simulink model "GTA_PCMFirmware"  (Simulink 7.8)
settings: Solver=FixedStepDiscrete  StartTime=0.0  StopTime=10.0  RelTol=1e-3
PreLoadFcn:
  | try, eval([bdroot '_setup']); catch, eval('model_setup', ''); end
InitFcn:
  | try, eval([bdroot '_setup']); catch, eval('model_setup', ''); end
undefined symbols (not defined in the file): fndFwd, fndNeut, fndRev, FWDlockout, GCM, keySwIgn2, motohawk_build_version, motohawk_trunc_name, motohawk_vardec_path, REVlockout
libraries: MotoHawk_lib x313, simulink x47, GTA_Library x13
(part 4 of 7)

== system GTA_PCMFirmware/Function/1 Inputs and Paramaters/CAN/ Motor Controller/TemperatureWarnFB ==
  note: TempWarnFdbkOK
  In1 : Inport
  Bus Creator : BusCreator
  Bus Selector : BusSelector  OutputSignals=CANTimeout
  Constant : Constant  Value=0  OutDataTypeStr=single
  Constant1 : Constant  Value=0  OutDataTypeStr=single
  Constant2 : Constant  Value=0  OutDataTypeStr=uint16
  Read CAN Message : MotoHawk_lib/CAN Blocks/Read CAN Message  nam='Isolated_CAN'  bus=-2  msg=CANMSG_TempWarnFB  queue=1  slot=''  valid=off  stale=on  labelwires=off
  Relational Operator : RelationalOperator  OutDataTypeStr=boolean
  Signal Specification : SignalSpecification  OutDataTypeStr=single
  Signal Specification1 : SignalSpecification  OutDataTypeStr=single
  Signal Specification2 : SignalSpecification  OutDataTypeStr=uint16
  Subsystem : GTA_Library/Subsystem
  Subsystem1 : GTA_Library/Subsystem
  Subsystem2 : GTA_Library/Subsystem
  motohawk_override_abs : MotoHawk_lib/Calibration & Probing Blocks/motohawk_override_abs  parent_name='WarningFlags'  parent_val=0  show_more=off  name_source=Use Parameter  parent_read_level=1  parent_override_level=1  view_as=Number  enum_struct={'Disabled', 'Enabled'}  use_help_units=off  parent_help=''  parent_units=''  use_min_max=off  parent_min=-inf  parent_max=inf  use_precision=off  parent_precision=''  parent_gain=1  parent_offset=0  parent_exp=1  use_mototune_group=off  parent_group=motohawk_vardec_path(gcb)
  motohawk_override_abs1 : MotoHawk_lib/Calibration & Probing Blocks/motohawk_override_abs  parent_name='MotorTemp'  parent_val=0  show_more=off  name_source=Use Parameter  parent_read_level=1  parent_override_level=1  view_as=Number  enum_struct={'Disabled', 'Enabled'}  use_help_units=off  parent_help=''  parent_units=''  use_min_max=off  parent_min=-inf  parent_max=inf  use_precision=off  parent_precision=''  parent_gain=1  parent_offset=0  parent_exp=1  use_mototune_group=off  parent_group=motohawk_vardec_path(gcb)
  motohawk_override_abs2 : MotoHawk_lib/Calibration & Probing Blocks/motohawk_override_abs  parent_name='HeatSinkTemp'  parent_val=0  show_more=off  name_source=Use Parameter  parent_read_level=1  parent_override_level=1  view_as=Number  enum_struct={'Disabled', 'Enabled'}  use_help_units=off  parent_help=''  parent_units=''  use_min_max=off  parent_min=-inf  parent_max=inf  use_precision=off  parent_precision=''  parent_gain=1  parent_offset=0  parent_exp=1  use_mototune_group=off  parent_group=motohawk_vardec_path(gcb)
  motohawk_probe1 : MotoHawk_lib/Calibration & Probing Blocks/motohawk_probe  nam='WarningFlags'  show_more=off  name_source=Use Parameter  read_level=1  view_as=Number  enum_struct={'Disabled', 'Enabled'}  vector_style=Wide Row  use_help_units=off  help=''  units=''  use_header_enum=off  row_header_enum={}  col_header_enum={}  use_min_max=off  min_val=-inf  max_val=inf  use_precision=off  precision=''  gain=1  offset=0  exp=1  use_mototune_group=off  mototune_group=motohawk_vardec_path(gcb)
  motohawk_probe2 : MotoHawk_lib/Calibration & Probing Blocks/motohawk_probe  nam='MotorTemp'  show_more=off  name_source=Use Parameter  read_level=1  view_as=Number  enum_struct={'Disabled', 'Enabled'}  vector_style=Wide Row  use_help_units=off  help=''  units=''  use_header_enum=off  row_header_enum={}  col_header_enum={}  use_min_max=off  min_val=-inf  max_val=inf  use_precision=off  precision=''  gain=1  offset=0  exp=1  use_mototune_group=off  mototune_group=motohawk_vardec_path(gcb)
  motohawk_probe3 : MotoHawk_lib/Calibration & Probing Blocks/motohawk_probe  nam='HeatSinkTemp'  show_more=off  name_source=Use Parameter  read_level=1  view_as=Number  enum_struct={'Disabled', 'Enabled'}  vector_style=Wide Row  use_help_units=off  help=''  units=''  use_header_enum=off  row_header_enum={}  col_header_enum={}  use_min_max=off  min_val=-inf  max_val=inf  use_precision=off  precision=''  gain=1  offset=0  exp=1  use_mototune_group=off  mototune_group=motohawk_vardec_path(gcb)
  KinTempWarn : Outport
  wires:
  In1/1 -> Bus Selector/1
  Read CAN Message/1 -> Relational Operator/2
  Bus Selector/1 -> Relational Operator/1, Subsystem/1, Subsystem1/1, Subsystem2/1, Subsystem/2, Subsystem1/2, Subsystem2/2  "<CANTimeout>"
  Read CAN Message/2 -> Signal Specification1/1
  Read CAN Message/3 -> Signal Specification/1
  Read CAN Message/4 -> Signal Specification2/1
  Signal Specification2/1 -> Subsystem2/3
  Signal Specification/1 -> Subsystem1/3
  Signal Specification1/1 -> Subsystem/3
  Constant/1 -> Subsystem/4
  Constant2/1 -> Subsystem2/4
  Constant1/1 -> Subsystem1/4
  Subsystem/1 -> motohawk_override_abs2/1, motohawk_probe3/1
  Subsystem1/1 -> motohawk_override_abs1/1, motohawk_probe2/1
  Subsystem2/1 -> motohawk_override_abs/1, motohawk_probe1/1
  motohawk_override_abs/1 -> Bus Creator/4  "WarningFlags"
  Relational Operator/1 -> Bus Creator/1
  motohawk_override_abs2/1 -> Bus Creator/2  "HeatSinkTemp"
  motohawk_override_abs1/1 -> Bus Creator/3  "MotorTemp"
  Bus Creator/1 -> KinTempWarn/1

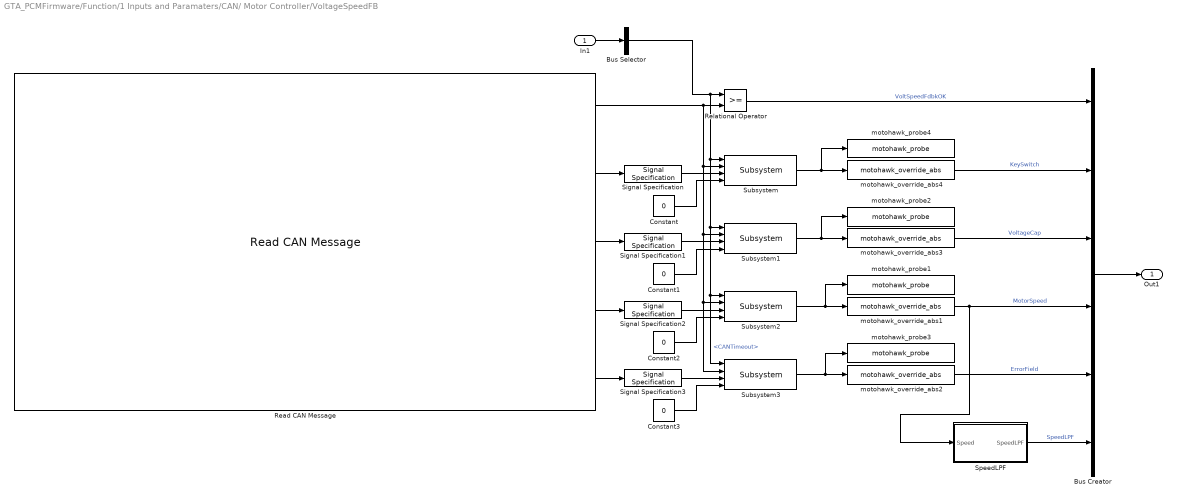
== system GTA_PCMFirmware/Function/1 Inputs and Paramaters/CAN/ Motor Controller/VoltageSpeedFB ==
  In1 : Inport
  Bus Creator : BusCreator  Inputs=6
  Bus Selector : BusSelector  OutputSignals=CANTimeout
  Constant : Constant  Value=0  OutDataTypeStr=single
  Constant1 : Constant  Value=0  OutDataTypeStr=single
  Constant2 : Constant  Value=0  OutDataTypeStr=single
  Constant3 : Constant  Value=0  OutDataTypeStr=uint16
  Read CAN Message : MotoHawk_lib/CAN Blocks/Read CAN Message  nam='Isolated_CAN'  bus=-2  msg=CANMSG_VoltSpeedFB  queue=1  slot=''  valid=off  stale=on  labelwires=off
  Relational Operator : RelationalOperator  OutDataTypeStr=boolean
  Signal Specification : SignalSpecification  OutDataTypeStr=single
  Signal Specification1 : SignalSpecification  OutDataTypeStr=single
  Signal Specification2 : SignalSpecification  OutDataTypeStr=single
  Signal Specification3 : SignalSpecification  OutDataTypeStr=uint16
  SpeedLPF : Subsystem
  Subsystem{,1..3} (4 alike) : GTA_Library/Subsystem
  motohawk_override_abs1 : MotoHawk_lib/Calibration & Probing Blocks/motohawk_override_abs  parent_name='SpeedFiltered'  parent_val=0  show_more=off  name_source=Use Parameter  parent_read_level=1  parent_override_level=1  view_as=Number  enum_struct={'Disabled', 'Enabled'}  use_help_units=off  parent_help=''  parent_units=''  use_min_max=off  parent_min=-inf  parent_max=inf  use_precision=off  parent_precision=''  parent_gain=1  parent_offset=0  parent_exp=1  use_mototune_group=off  parent_group=motohawk_vardec_path(gcb)
  motohawk_override_abs2 : MotoHawk_lib/Calibration & Probing Blocks/motohawk_override_abs  parent_name='ErrorField'  parent_val=0  show_more=off  name_source=Use Parameter  parent_read_level=1  parent_override_level=1  view_as=Number  enum_struct={'Disabled', 'Enabled'}  use_help_units=off  parent_help=''  parent_units=''  use_min_max=off  parent_min=-inf  parent_max=inf  use_precision=off  parent_precision=''  parent_gain=1  parent_offset=0  parent_exp=1  use_mototune_group=off  parent_group=motohawk_vardec_path(gcb)
  motohawk_override_abs3 : MotoHawk_lib/Calibration & Probing Blocks/motohawk_override_abs  parent_name='Voltage_Cap'  parent_val=0  show_more=off  name_source=Use Parameter  parent_read_level=1  parent_override_level=1  view_as=Number  enum_struct={'Disabled', 'Enabled'}  use_help_units=off  parent_help=''  parent_units=''  use_min_max=off  parent_min=-inf  parent_max=inf  use_precision=off  parent_precision=''  parent_gain=1  parent_offset=0  parent_exp=1  use_mototune_group=off  parent_group=motohawk_vardec_path(gcb)
  motohawk_override_abs4 : MotoHawk_lib/Calibration & Probing Blocks/motohawk_override_abs  parent_name='KeySwVoltage'  parent_val=0  show_more=off  name_source=Use Parameter  parent_read_level=1  parent_override_level=1  view_as=Number  enum_struct={'Disabled', 'Enabled'}  use_help_units=off  parent_help=''  parent_units=''  use_min_max=off  parent_min=-inf  parent_max=inf  use_precision=off  parent_precision=''  parent_gain=1  parent_offset=0  parent_exp=1  use_mototune_group=off  parent_group=motohawk_vardec_path(gcb)
  motohawk_probe1 : MotoHawk_lib/Calibration & Probing Blocks/motohawk_probe  nam='SpeedFiltered'  show_more=off  name_source=Use Parameter  read_level=1  view_as=Number  enum_struct={'Disabled', 'Enabled'}  vector_style=Wide Row  use_help_units=off  help=''  units=''  use_header_enum=off  row_header_enum={}  col_header_enum={}  use_min_max=off  min_val=-inf  max_val=inf  use_precision=off  precision=''  gain=1  offset=0  exp=1  use_mototune_group=off  mototune_group=motohawk_vardec_path(gcb)
  motohawk_probe2 : MotoHawk_lib/Calibration & Probing Blocks/motohawk_probe  nam='Voltage_Cap'  show_more=off  name_source=Use Parameter  read_level=1  view_as=Number  enum_struct={'Disabled', 'Enabled'}  vector_style=Wide Row  use_help_units=off  help=''  units=''  use_header_enum=off  row_header_enum={}  col_header_enum={}  use_min_max=off  min_val=-inf  max_val=inf  use_precision=off  precision=''  gain=1  offset=0  exp=1  use_mototune_group=off  mototune_group=motohawk_vardec_path(gcb)
  motohawk_probe3 : MotoHawk_lib/Calibration & Probing Blocks/motohawk_probe  nam='ErrorField'  show_more=off  name_source=Use Parameter  read_level=1  view_as=Number  enum_struct={'Disabled', 'Enabled'}  vector_style=Wide Row  use_help_units=off  help=''  units=''  use_header_enum=off  row_header_enum={}  col_header_enum={}  use_min_max=off  min_val=-inf  max_val=inf  use_precision=off  precision=''  gain=1  offset=0  exp=1  use_mototune_group=off  mototune_group=motohawk_vardec_path(gcb)
  motohawk_probe4 : MotoHawk_lib/Calibration & Probing Blocks/motohawk_probe  nam='KeySwVoltage'  show_more=off  name_source=Use Parameter  read_level=1  view_as=Number  enum_struct={'Disabled', 'Enabled'}  vector_style=Wide Row  use_help_units=off  help=''  units=''  use_header_enum=off  row_header_enum={}  col_header_enum={}  use_min_max=off  min_val=-inf  max_val=inf  use_precision=off  precision=''  gain=1  offset=0  exp=1  use_mototune_group=off  mototune_group=motohawk_vardec_path(gcb)
  Out1 : Outport
  wires:
  In1/1 -> Bus Selector/1
  Read CAN Message/1 -> Relational Operator/2, Subsystem/2, Subsystem1/2, Subsystem2/2, Subsystem3/2
  Bus Selector/1 -> Relational Operator/1, Subsystem/1, Subsystem1/1, Subsystem2/1, Subsystem3/1  "<CANTimeout>"
  Read CAN Message/2 -> Signal Specification/1
  Read CAN Message/5 -> Signal Specification3/1
  Read CAN Message/4 -> Signal Specification2/1
  Read CAN Message/3 -> Signal Specification1/1
  Constant/1 -> Subsystem/4
  Signal Specification/1 -> Subsystem/3
  Signal Specification1/1 -> Subsystem1/3
  Constant1/1 -> Subsystem1/4
  Signal Specification2/1 -> Subsystem2/3
  Constant2/1 -> Subsystem2/4
  Constant3/1 -> Subsystem3/4
  Signal Specification3/1 -> Subsystem3/3
  Subsystem/1 -> motohawk_override_abs4/1, motohawk_probe4/1
  Subsystem1/1 -> motohawk_override_abs3/1, motohawk_probe2/1
  Subsystem2/1 -> motohawk_override_abs1/1, motohawk_probe1/1
  Subsystem3/1 -> motohawk_override_abs2/1, motohawk_probe3/1
  motohawk_override_abs2/1 -> Bus Creator/5  "ErrorField"
  Relational Operator/1 -> Bus Creator/1  "VoltSpeedFdbkOK"
  motohawk_override_abs1/1 -> Bus Creator/4, SpeedLPF/1(Speed)  "MotorSpeed"
  motohawk_override_abs3/1 -> Bus Creator/3  "VoltageCap"
  motohawk_override_abs4/1 -> Bus Creator/2  "KeySwitch"
  SpeedLPF/1(SpeedLPF) -> Bus Creator/6  "SpeedLPF"
  Bus Creator/1 -> Out1/1

== system GTA_PCMFirmware/Function/1 Inputs and Paramaters/CAN/ Motor Controller/Watchdog ==
  In1 : Inport
  Bus Creator : BusCreator  Inputs=2
  Bus Selector : BusSelector  OutputSignals=CANTimeout
  Constant3 : Constant  Value=0  OutDataTypeStr=uint16
  Read CAN Message : MotoHawk_lib/CAN Blocks/Read CAN Message  nam='Isolated_CAN'  bus=-2  msg=CANMSG_Watchdog  queue=1  slot=''  valid=off  stale=on  labelwires=off
  Relational Operator : RelationalOperator  OutDataTypeStr=boolean
  Signal Specification3 : SignalSpecification  OutDataTypeStr=uint16
  Subsystem : GTA_Library/Subsystem
  motohawk_override_abs2 : MotoHawk_lib/Calibration & Probing Blocks/motohawk_override_abs  parent_name='WDcounter'  parent_val=0  show_more=off  name_source=Use Parameter  parent_read_level=1  parent_override_level=1  view_as=Number  enum_struct={'Disabled', 'Enabled'}  use_help_units=off  parent_help=''  parent_units=''  use_min_max=off  parent_min=-inf  parent_max=inf  use_precision=off  parent_precision=''  parent_gain=1  parent_offset=0  parent_exp=1  use_mototune_group=off  parent_group=motohawk_vardec_path(gcb)
  motohawk_probe3 : MotoHawk_lib/Calibration & Probing Blocks/motohawk_probe  nam='WDcounter'  show_more=off  name_source=Use Parameter  read_level=1  view_as=Number  enum_struct={'Disabled', 'Enabled'}  vector_style=Wide Row  use_help_units=off  help=''  units=''  use_header_enum=off  row_header_enum={}  col_header_enum={}  use_min_max=off  min_val=-inf  max_val=inf  use_precision=off  precision=''  gain=1  offset=0  exp=1  use_mototune_group=off  mototune_group=motohawk_vardec_path(gcb)
  KinWatchdog : Outport
  wires:
  In1/1 -> Bus Selector/1
  Constant3/1 -> Subsystem/4
  Signal Specification3/1 -> Subsystem/3
  Read CAN Message/2 -> Signal Specification3/1
  Read CAN Message/1 -> Relational Operator/2, Subsystem/2
  Bus Selector/1 -> Relational Operator/1, Subsystem/1  "<CANTimeout>"
  Relational Operator/1 -> Bus Creator/1  "WatchdogCANok"
  Subsystem/1 -> motohawk_override_abs2/1, motohawk_probe3/1
  motohawk_override_abs2/1 -> Bus Creator/2  "WDcounter"
  Bus Creator/1 -> KinWatchdog/1

== system GTA_PCMFirmware/Function/1 Inputs and Paramaters/CAN/BMS/  Current Sensor ==
  CAN Params : Inport
  Bus Creator : BusCreator  Inputs=6
  Bus Selector : BusSelector  OutputSignals=CANTimeout,MinSOC
  Read CAN Message : MotoHawk_lib/CAN Blocks/Read CAN Message  nam='BMS_CAN'  bus=-2  msg=CANMSG_FluxPowerCurrentSensor  queue=1  slot=''  valid=off  stale=on  labelwires=off
  Relational Operator : RelationalOperator  OutDataTypeStr=boolean
  Signal Specification{,1..3} (4 alike) : SignalSpecification  OutDataTypeStr=single
  UserSOC : Subsystem
  motohawk_override_abs : MotoHawk_lib/Calibration & Probing Blocks/motohawk_override_abs  parent_name='CurrentSensor_Current'  parent_val=0  show_more=off  name_source=Use Parameter  parent_read_level=1  parent_override_level=1  view_as=Number  enum_struct={'Disabled', 'Enabled'}  use_help_units=off  parent_help=''  parent_units=''  use_min_max=off  parent_min=-inf  parent_max=inf  use_precision=off  parent_precision=''  parent_gain=1  parent_offset=0  parent_exp=1  use_mototune_group=off  parent_group=motohawk_vardec_path(gcb)
  motohawk_override_abs1 : MotoHawk_lib/Calibration & Probing Blocks/motohawk_override_abs  parent_name='CurrentSensor_SOC'  parent_val=0  show_more=off  name_source=Use Parameter  parent_read_level=1  parent_override_level=1  view_as=Number  enum_struct={'Disabled', 'Enabled'}  use_help_units=off  parent_help=''  parent_units=''  use_min_max=off  parent_min=-inf  parent_max=inf  use_precision=off  parent_precision=''  parent_gain=1  parent_offset=0  parent_exp=1  use_mototune_group=off  parent_group=motohawk_vardec_path(gcb)
  motohawk_override_abs2 : MotoHawk_lib/Calibration & Probing Blocks/motohawk_override_abs  parent_name='CurrentSensor_Temperature'  parent_val=0  show_more=off  name_source=Use Parameter  parent_read_level=1  parent_override_level=1  view_as=Number  enum_struct={'Disabled', 'Enabled'}  use_help_units=off  parent_help=''  parent_units=''  use_min_max=off  parent_min=-inf  parent_max=inf  use_precision=off  parent_precision=''  parent_gain=1  parent_offset=0  parent_exp=1  use_mototune_group=off  parent_group=motohawk_vardec_path(gcb)
  motohawk_override_abs3 : MotoHawk_lib/Calibration & Probing Blocks/motohawk_override_abs  parent_name='CurrentSensor_AmpHours'  parent_val=0  show_more=off  name_source=Use Parameter  parent_read_level=1  parent_override_level=1  view_as=Number  enum_struct={'Disabled', 'Enabled'}  use_help_units=off  parent_help=''  parent_units=''  use_min_max=off  parent_min=-inf  parent_max=inf  use_precision=off  parent_precision=''  parent_gain=1  parent_offset=0  parent_exp=1  use_mototune_group=off  parent_group=motohawk_vardec_path(gcb)
  motohawk_probe : MotoHawk_lib/Calibration & Probing Blocks/motohawk_probe  nam='CurrentSensor_Current'  show_more=off  name_source=Use Parameter  read_level=1  view_as=Number  enum_struct={'Disabled', 'Enabled'}  vector_style=Wide Row  use_help_units=off  help=''  units=''  use_header_enum=off  row_header_enum={}  col_header_enum={}  use_min_max=off  min_val=-inf  max_val=inf  use_precision=off  precision=''  gain=1  offset=0  exp=1  use_mototune_group=off  mototune_group=motohawk_vardec_path(gcb)
  motohawk_probe1 : MotoHawk_lib/Calibration & Probing Blocks/motohawk_probe  nam='CurrentSensor_SOC'  show_more=off  name_source=Use Parameter  read_level=1  view_as=Number  enum_struct={'Disabled', 'Enabled'}  vector_style=Wide Row  use_help_units=off  help=''  units=''  use_header_enum=off  row_header_enum={}  col_header_enum={}  use_min_max=off  min_val=-inf  max_val=inf  use_precision=off  precision=''  gain=1  offset=0  exp=1  use_mototune_group=off  mototune_group=motohawk_vardec_path(gcb)
  motohawk_probe2 : MotoHawk_lib/Calibration & Probing Blocks/motohawk_probe  nam='CurrentSensor_Temperature'  show_more=off  name_source=Use Parameter  read_level=1  view_as=Number  enum_struct={'Disabled', 'Enabled'}  vector_style=Wide Row  use_help_units=off  help=''  units=''  use_header_enum=off  row_header_enum={}  col_header_enum={}  use_min_max=off  min_val=-inf  max_val=inf  use_precision=off  precision=''  gain=1  offset=0  exp=1  use_mototune_group=off  mototune_group=motohawk_vardec_path(gcb)
  motohawk_probe3 : MotoHawk_lib/Calibration & Probing Blocks/motohawk_probe  nam='CurrentSensor_AmpHours'  show_more=off  name_source=Use Parameter  read_level=1  view_as=Number  enum_struct={'Disabled', 'Enabled'}  vector_style=Wide Row  use_help_units=off  help=''  units=''  use_header_enum=off  row_header_enum={}  col_header_enum={}  use_min_max=off  min_val=-inf  max_val=inf  use_precision=off  precision=''  gain=1  offset=0  exp=1  use_mototune_group=off  mototune_group=motohawk_vardec_path(gcb)
  Current Sensor : Outport
  wires:
  Read CAN Message/1 -> Relational Operator/2
  CAN Params/1 -> Bus Selector/1
  Bus Selector/1 -> Relational Operator/1  "<CANTimeout>"
  Read CAN Message/2 -> Signal Specification/1
  Read CAN Message/3 -> Signal Specification1/1
  Read CAN Message/4 -> Signal Specification2/1
  Read CAN Message/5 -> Signal Specification3/1
  Signal Specification/1 -> motohawk_override_abs/1, motohawk_probe/1
  Signal Specification1/1 -> motohawk_override_abs1/1, motohawk_probe1/1
  Signal Specification2/1 -> motohawk_override_abs2/1, motohawk_probe2/1
  Signal Specification3/1 -> motohawk_override_abs3/1, motohawk_probe3/1
  motohawk_override_abs3/1 -> Bus Creator/5  "csAmpHours"
  motohawk_override_abs2/1 -> Bus Creator/4  "csTemperature"
  motohawk_override_abs1/1 -> Bus Creator/3, UserSOC/1(csSOC)  "csSOC"
  motohawk_override_abs/1 -> Bus Creator/2  "csCurrent"
  Relational Operator/1 -> Bus Creator/1  "csCANok"
  Bus Creator/1 -> Current Sensor/1
  Bus Selector/2 -> UserSOC/2(MinSOC)  "<MinSOC>"
  UserSOC/1(UserSOC) -> Bus Creator/6  "UserSOC"

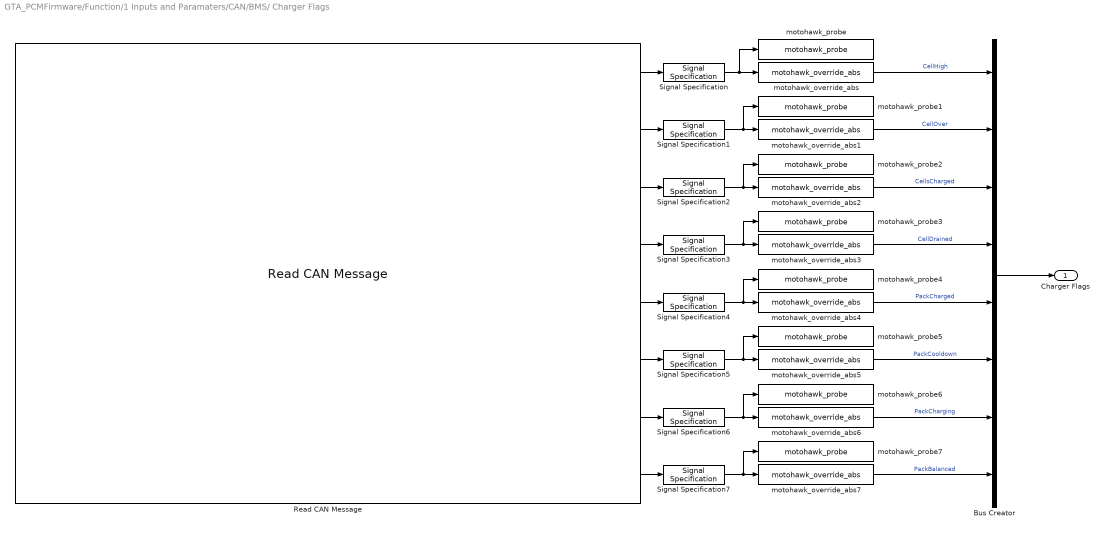
== system GTA_PCMFirmware/Function/1 Inputs and Paramaters/CAN/BMS/ Charger Flags ==
  Bus Creator : BusCreator  Inputs=8
  Read CAN Message : MotoHawk_lib/CAN Blocks/Read CAN Message  nam='BMS_CAN'  bus=-2  msg=CANMSG_FluxPowerCSChargeFlags  queue=1  slot=''  valid=off  stale=off  labelwires=off
  Signal Specification{,1..7} (8 alike) : SignalSpecification  OutDataTypeStr=boolean
  motohawk_override_abs : MotoHawk_lib/Calibration & Probing Blocks/motohawk_override_abs  parent_name='CellHigh'  parent_val=0  show_more=off  name_source=Use Parameter  parent_read_level=1  parent_override_level=1  view_as=Number  enum_struct={'Disabled', 'Enabled'}  use_help_units=off  parent_help=''  parent_units=''  use_min_max=off  parent_min=-inf  parent_max=inf  use_precision=off  parent_precision=''  parent_gain=1  parent_offset=0  parent_exp=1  use_mototune_group=off  parent_group=motohawk_vardec_path(gcb)
  motohawk_override_abs1 : MotoHawk_lib/Calibration & Probing Blocks/motohawk_override_abs  parent_name='CellOver'  parent_val=0  show_more=off  name_source=Use Parameter  parent_read_level=1  parent_override_level=1  view_as=Number  enum_struct={'Disabled', 'Enabled'}  use_help_units=off  parent_help=''  parent_units=''  use_min_max=off  parent_min=-inf  parent_max=inf  use_precision=off  parent_precision=''  parent_gain=1  parent_offset=0  parent_exp=1  use_mototune_group=off  parent_group=motohawk_vardec_path(gcb)
  motohawk_override_abs2 : MotoHawk_lib/Calibration & Probing Blocks/motohawk_override_abs  parent_name='CellsCharged'  parent_val=0  show_more=off  name_source=Use Parameter  parent_read_level=1  parent_override_level=1  view_as=Number  enum_struct={'Disabled', 'Enabled'}  use_help_units=off  parent_help=''  parent_units=''  use_min_max=off  parent_min=-inf  parent_max=inf  use_precision=off  parent_precision=''  parent_gain=1  parent_offset=0  parent_exp=1  use_mototune_group=off  parent_group=motohawk_vardec_path(gcb)
  motohawk_override_abs3 : MotoHawk_lib/Calibration & Probing Blocks/motohawk_override_abs  parent_name='CellDrained'  parent_val=0  show_more=off  name_source=Use Parameter  parent_read_level=1  parent_override_level=1  view_as=Number  enum_struct={'Disabled', 'Enabled'}  use_help_units=off  parent_help=''  parent_units=''  use_min_max=off  parent_min=-inf  parent_max=inf  use_precision=off  parent_precision=''  parent_gain=1  parent_offset=0  parent_exp=1  use_mototune_group=off  parent_group=motohawk_vardec_path(gcb)
  motohawk_override_abs4 : MotoHawk_lib/Calibration & Probing Blocks/motohawk_override_abs  parent_name='PackCharged'  parent_val=0  show_more=off  name_source=Use Parameter  parent_read_level=1  parent_override_level=1  view_as=Number  enum_struct={'Disabled', 'Enabled'}  use_help_units=off  parent_help=''  parent_units=''  use_min_max=off  parent_min=-inf  parent_max=inf  use_precision=off  parent_precision=''  parent_gain=1  parent_offset=0  parent_exp=1  use_mototune_group=off  parent_group=motohawk_vardec_path(gcb)
  motohawk_override_abs5 : MotoHawk_lib/Calibration & Probing Blocks/motohawk_override_abs  parent_name='PackCooldown'  parent_val=0  show_more=off  name_source=Use Parameter  parent_read_level=1  parent_override_level=1  view_as=Number  enum_struct={'Disabled', 'Enabled'}  use_help_units=off  parent_help=''  parent_units=''  use_min_max=off  parent_min=-inf  parent_max=inf  use_precision=off  parent_precision=''  parent_gain=1  parent_offset=0  parent_exp=1  use_mototune_group=off  parent_group=motohawk_vardec_path(gcb)
  motohawk_override_abs6 : MotoHawk_lib/Calibration & Probing Blocks/motohawk_override_abs  parent_name='PackCharging'  parent_val=0  show_more=off  name_source=Use Parameter  parent_read_level=1  parent_override_level=1  view_as=Number  enum_struct={'Disabled', 'Enabled'}  use_help_units=off  parent_help=''  parent_units=''  use_min_max=off  parent_min=-inf  parent_max=inf  use_precision=off  parent_precision=''  parent_gain=1  parent_offset=0  parent_exp=1  use_mototune_group=off  parent_group=motohawk_vardec_path(gcb)
  motohawk_override_abs7 : MotoHawk_lib/Calibration & Probing Blocks/motohawk_override_abs  parent_name='PackBalanced'  parent_val=0  show_more=off  name_source=Use Parameter  parent_read_level=1  parent_override_level=1  view_as=Number  enum_struct={'Disabled', 'Enabled'}  use_help_units=off  parent_help=''  parent_units=''  use_min_max=off  parent_min=-inf  parent_max=inf  use_precision=off  parent_precision=''  parent_gain=1  parent_offset=0  parent_exp=1  use_mototune_group=off  parent_group=motohawk_vardec_path(gcb)
  motohawk_probe : MotoHawk_lib/Calibration & Probing Blocks/motohawk_probe  nam='CellHigh'  show_more=off  name_source=Use Parameter  read_level=1  view_as=Number  enum_struct={'Disabled', 'Enabled'}  vector_style=Wide Row  use_help_units=off  help=''  units=''  use_header_enum=off  row_header_enum={}  col_header_enum={}  use_min_max=off  min_val=-inf  max_val=inf  use_precision=off  precision=''  gain=1  offset=0  exp=1  use_mototune_group=off  mototune_group=motohawk_vardec_path(gcb)
  motohawk_probe1 : MotoHawk_lib/Calibration & Probing Blocks/motohawk_probe  nam='CellOver'  show_more=off  name_source=Use Parameter  read_level=1  view_as=Number  enum_struct={'Disabled', 'Enabled'}  vector_style=Wide Row  use_help_units=off  help=''  units=''  use_header_enum=off  row_header_enum={}  col_header_enum={}  use_min_max=off  min_val=-inf  max_val=inf  use_precision=off  precision=''  gain=1  offset=0  exp=1  use_mototune_group=off  mototune_group=motohawk_vardec_path(gcb)
  motohawk_probe2 : MotoHawk_lib/Calibration & Probing Blocks/motohawk_probe  nam='CellsCharged'  show_more=off  name_source=Use Parameter  read_level=1  view_as=Number  enum_struct={'Disabled', 'Enabled'}  vector_style=Wide Row  use_help_units=off  help=''  units=''  use_header_enum=off  row_header_enum={}  col_header_enum={}  use_min_max=off  min_val=-inf  max_val=inf  use_precision=off  precision=''  gain=1  offset=0  exp=1  use_mototune_group=off  mototune_group=motohawk_vardec_path(gcb)
  motohawk_probe3 : MotoHawk_lib/Calibration & Probing Blocks/motohawk_probe  nam='CellDrained'  show_more=off  name_source=Use Parameter  read_level=1  view_as=Number  enum_struct={'Disabled', 'Enabled'}  vector_style=Wide Row  use_help_units=off  help=''  units=''  use_header_enum=off  row_header_enum={}  col_header_enum={}  use_min_max=off  min_val=-inf  max_val=inf  use_precision=off  precision=''  gain=1  offset=0  exp=1  use_mototune_group=off  mototune_group=motohawk_vardec_path(gcb)
  motohawk_probe4 : MotoHawk_lib/Calibration & Probing Blocks/motohawk_probe  nam='PackCharged'  show_more=off  name_source=Use Parameter  read_level=1  view_as=Number  enum_struct={'Disabled', 'Enabled'}  vector_style=Wide Row  use_help_units=off  help=''  units=''  use_header_enum=off  row_header_enum={}  col_header_enum={}  use_min_max=off  min_val=-inf  max_val=inf  use_precision=off  precision=''  gain=1  offset=0  exp=1  use_mototune_group=off  mototune_group=motohawk_vardec_path(gcb)
  motohawk_probe5 : MotoHawk_lib/Calibration & Probing Blocks/motohawk_probe  nam='PackCooldown'  show_more=off  name_source=Use Parameter  read_level=1  view_as=Number  enum_struct={'Disabled', 'Enabled'}  vector_style=Wide Row  use_help_units=off  help=''  units=''  use_header_enum=off  row_header_enum={}  col_header_enum={}  use_min_max=off  min_val=-inf  max_val=inf  use_precision=off  precision=''  gain=1  offset=0  exp=1  use_mototune_group=off  mototune_group=motohawk_vardec_path(gcb)
  motohawk_probe6 : MotoHawk_lib/Calibration & Probing Blocks/motohawk_probe  nam='PackCharging'  show_more=off  name_source=Use Parameter  read_level=1  view_as=Number  enum_struct={'Disabled', 'Enabled'}  vector_style=Wide Row  use_help_units=off  help=''  units=''  use_header_enum=off  row_header_enum={}  col_header_enum={}  use_min_max=off  min_val=-inf  max_val=inf  use_precision=off  precision=''  gain=1  offset=0  exp=1  use_mototune_group=off  mototune_group=motohawk_vardec_path(gcb)
  motohawk_probe7 : MotoHawk_lib/Calibration & Probing Blocks/motohawk_probe  nam='PackBalanced'  show_more=off  name_source=Use Parameter  read_level=1  view_as=Number  enum_struct={'Disabled', 'Enabled'}  vector_style=Wide Row  use_help_units=off  help=''  units=''  use_header_enum=off  row_header_enum={}  col_header_enum={}  use_min_max=off  min_val=-inf  max_val=inf  use_precision=off  precision=''  gain=1  offset=0  exp=1  use_mototune_group=off  mototune_group=motohawk_vardec_path(gcb)
  Charger Flags : Outport
  wires:
  Read CAN Message/1 -> Signal Specification/1
  Read CAN Message/2 -> Signal Specification1/1
  Read CAN Message/3 -> Signal Specification2/1
  Read CAN Message/4 -> Signal Specification3/1
  Read CAN Message/5 -> Signal Specification4/1
  Read CAN Message/6 -> Signal Specification5/1
  Read CAN Message/7 -> Signal Specification6/1
  Read CAN Message/8 -> Signal Specification7/1
  Signal Specification/1 -> motohawk_override_abs/1, motohawk_probe/1
  Signal Specification1/1 -> motohawk_override_abs1/1, motohawk_probe1/1
  Signal Specification2/1 -> motohawk_override_abs2/1, motohawk_probe2/1
  Signal Specification3/1 -> motohawk_override_abs3/1, motohawk_probe3/1
  Signal Specification4/1 -> motohawk_override_abs4/1, motohawk_probe4/1
  Signal Specification5/1 -> motohawk_override_abs5/1, motohawk_probe5/1
  Signal Specification6/1 -> motohawk_override_abs6/1, motohawk_probe6/1
  Signal Specification7/1 -> motohawk_override_abs7/1, motohawk_probe7/1
  motohawk_override_abs/1 -> Bus Creator/1  "CellHigh"
  motohawk_override_abs1/1 -> Bus Creator/2  "CellOver"
  motohawk_override_abs2/1 -> Bus Creator/3  "CellsCharged"
  motohawk_override_abs3/1 -> Bus Creator/4  "CellDrained"
  motohawk_override_abs4/1 -> Bus Creator/5  "PackCharged"
  motohawk_override_abs5/1 -> Bus Creator/6  "PackCooldown"
  motohawk_override_abs6/1 -> Bus Creator/7  "PackCharging"
  motohawk_override_abs7/1 -> Bus Creator/8  "PackBalanced"
  Bus Creator/1 -> Charger Flags/1

== system GTA_PCMFirmware/Function/1 Inputs and Paramaters/CAN/BMS/Cell Information ==
  Bus Creator : BusCreator  Inputs=5
  Read CAN Message : MotoHawk_lib/CAN Blocks/Read CAN Message  nam='BMS_CAN'  bus=-2  msg=CANMSG_FluxPowerCSCellInfo  queue=1  slot=''  valid=off  stale=off  labelwires=off
  Signal Specification : SignalSpecification  OutDataTypeStr=uint8
  Signal Specification1 : SignalSpecification  OutDataTypeStr=single
  Signal Specification2 : SignalSpecification  OutDataTypeStr=uint8
  Signal Specification3 : SignalSpecification  OutDataTypeStr=single
  Signal Specification4 : SignalSpecification  OutDataTypeStr=single
  motohawk_override_abs : MotoHawk_lib/Calibration & Probing Blocks/motohawk_override_abs  parent_name='HighCell'  parent_val=0  show_more=off  name_source=Use Parameter  parent_read_level=1  parent_override_level=1  view_as=Number  enum_struct={'Disabled', 'Enabled'}  use_help_units=off  parent_help=''  parent_units=''  use_min_max=off  parent_min=-inf  parent_max=inf  use_precision=off  parent_precision=''  parent_gain=1  parent_offset=0  parent_exp=1  use_mototune_group=off  parent_group=motohawk_vardec_path(gcb)
  motohawk_override_abs1 : MotoHawk_lib/Calibration & Probing Blocks/motohawk_override_abs  parent_name='HighCellValue'  parent_val=0  show_more=off  name_source=Use Parameter  parent_read_level=1  parent_override_level=1  view_as=Number  enum_struct={'Disabled', 'Enabled'}  use_help_units=off  parent_help=''  parent_units=''  use_min_max=off  parent_min=-inf  parent_max=inf  use_precision=off  parent_precision=''  parent_gain=1  parent_offset=0  parent_exp=1  use_mototune_group=off  parent_group=motohawk_vardec_path(gcb)
  motohawk_override_abs2 : MotoHawk_lib/Calibration & Probing Blocks/motohawk_override_abs  parent_name='LowCell'  parent_val=0  show_more=off  name_source=Use Parameter  parent_read_level=1  parent_override_level=1  view_as=Number  enum_struct={'Disabled', 'Enabled'}  use_help_units=off  parent_help=''  parent_units=''  use_min_max=off  parent_min=-inf  parent_max=inf  use_precision=off  parent_precision=''  parent_gain=1  parent_offset=0  parent_exp=1  use_mototune_group=off  parent_group=motohawk_vardec_path(gcb)
  motohawk_override_abs3 : MotoHawk_lib/Calibration & Probing Blocks/motohawk_override_abs  parent_name='LowCellValue'  parent_val=0  show_more=off  name_source=Use Parameter  parent_read_level=1  parent_override_level=1  view_as=Number  enum_struct={'Disabled', 'Enabled'}  use_help_units=off  parent_help=''  parent_units=''  use_min_max=off  parent_min=-inf  parent_max=inf  use_precision=off  parent_precision=''  parent_gain=1  parent_offset=0  parent_exp=1  use_mototune_group=off  parent_group=motohawk_vardec_path(gcb)
  motohawk_override_abs4 : MotoHawk_lib/Calibration & Probing Blocks/motohawk_override_abs  parent_name='PackVoltage'  parent_val=0  show_more=off  name_source=Use Parameter  parent_read_level=1  parent_override_level=1  view_as=Number  enum_struct={'Disabled', 'Enabled'}  use_help_units=off  parent_help=''  parent_units=''  use_min_max=off  parent_min=-inf  parent_max=inf  use_precision=off  parent_precision=''  parent_gain=1  parent_offset=0  parent_exp=1  use_mototune_group=off  parent_group=motohawk_vardec_path(gcb)
  motohawk_probe : MotoHawk_lib/Calibration & Probing Blocks/motohawk_probe  nam='HighCell'  show_more=off  name_source=Use Parameter  read_level=1  view_as=Number  enum_struct={'Disabled', 'Enabled'}  vector_style=Wide Row  use_help_units=off  help=''  units=''  use_header_enum=off  row_header_enum={}  col_header_enum={}  use_min_max=off  min_val=-inf  max_val=inf  use_precision=off  precision=''  gain=1  offset=0  exp=1  use_mototune_group=off  mototune_group=motohawk_vardec_path(gcb)
  motohawk_probe1 : MotoHawk_lib/Calibration & Probing Blocks/motohawk_probe  nam='HighCellValue'  show_more=off  name_source=Use Parameter  read_level=1  view_as=Number  enum_struct={'Disabled', 'Enabled'}  vector_style=Wide Row  use_help_units=off  help=''  units=''  use_header_enum=off  row_header_enum={}  col_header_enum={}  use_min_max=off  min_val=-inf  max_val=inf  use_precision=off  precision=''  gain=1  offset=0  exp=1  use_mototune_group=off  mototune_group=motohawk_vardec_path(gcb)
  motohawk_probe2 : MotoHawk_lib/Calibration & Probing Blocks/motohawk_probe  nam='LowCell'  show_more=off  name_source=Use Parameter  read_level=1  view_as=Number  enum_struct={'Disabled', 'Enabled'}  vector_style=Wide Row  use_help_units=off  help=''  units=''  use_header_enum=off  row_header_enum={}  col_header_enum={}  use_min_max=off  min_val=-inf  max_val=inf  use_precision=off  precision=''  gain=1  offset=0  exp=1  use_mototune_group=off  mototune_group=motohawk_vardec_path(gcb)
  motohawk_probe3 : MotoHawk_lib/Calibration & Probing Blocks/motohawk_probe  nam='LowCellValue'  show_more=off  name_source=Use Parameter  read_level=1  view_as=Number  enum_struct={'Disabled', 'Enabled'}  vector_style=Wide Row  use_help_units=off  help=''  units=''  use_header_enum=off  row_header_enum={}  col_header_enum={}  use_min_max=off  min_val=-inf  max_val=inf  use_precision=off  precision=''  gain=1  offset=0  exp=1  use_mototune_group=off  mototune_group=motohawk_vardec_path(gcb)
  motohawk_probe4 : MotoHawk_lib/Calibration & Probing Blocks/motohawk_probe  nam='PackVoltage'  show_more=off  name_source=Use Parameter  read_level=1  view_as=Number  enum_struct={'Disabled', 'Enabled'}  vector_style=Wide Row  use_help_units=off  help=''  units=''  use_header_enum=off  row_header_enum={}  col_header_enum={}  use_min_max=off  min_val=-inf  max_val=inf  use_precision=off  precision=''  gain=1  offset=0  exp=1  use_mototune_group=off  mototune_group=motohawk_vardec_path(gcb)
  Cell Info : Outport
  wires:
  Read CAN Message/1 -> Signal Specification/1
  Read CAN Message/2 -> Signal Specification1/1
  Read CAN Message/3 -> Signal Specification2/1
  Read CAN Message/4 -> Signal Specification3/1
  Read CAN Message/5 -> Signal Specification4/1
  Signal Specification/1 -> motohawk_override_abs/1, motohawk_probe/1
  Signal Specification1/1 -> motohawk_override_abs1/1, motohawk_probe1/1
  Signal Specification2/1 -> motohawk_override_abs2/1, motohawk_probe2/1
  Signal Specification3/1 -> motohawk_override_abs3/1, motohawk_probe3/1
  Signal Specification4/1 -> motohawk_override_abs4/1, motohawk_probe4/1
  motohawk_override_abs/1 -> Bus Creator/1  "HighCell"
  motohawk_override_abs4/1 -> Bus Creator/5  "PackVoltage"
  motohawk_override_abs3/1 -> Bus Creator/4  "LowCellValue"
  motohawk_override_abs2/1 -> Bus Creator/3  "LowCell"
  motohawk_override_abs1/1 -> Bus Creator/2  "HighCellValue"
  Bus Creator/1 -> Cell Info/1

== system GTA_PCMFirmware/Function/1 Inputs and Paramaters/CAN/BMS/Cell Temp ==
  Bus Creator : BusCreator  Inputs=2
  Read CAN Message : MotoHawk_lib/CAN Blocks/Read CAN Message  nam='BMS_CAN'  bus=-2  msg=CANMSG_FluxPowerCSCellTemp  queue=1  slot=''  valid=off  stale=off  labelwires=off
  Signal Specification : SignalSpecification  OutDataTypeStr=single
  Signal Specification1 : SignalSpecification  OutDataTypeStr=single
  motohawk_override_abs : MotoHawk_lib/Calibration & Probing Blocks/motohawk_override_abs  parent_name='HighCellTemp'  parent_val=0  show_more=off  name_source=Use Parameter  parent_read_level=1  parent_override_level=1  view_as=Number  enum_struct={'Disabled', 'Enabled'}  use_help_units=off  parent_help=''  parent_units=''  use_min_max=off  parent_min=-inf  parent_max=inf  use_precision=off  parent_precision=''  parent_gain=1  parent_offset=0  parent_exp=1  use_mototune_group=off  parent_group=motohawk_vardec_path(gcb)
  motohawk_override_abs1 : MotoHawk_lib/Calibration & Probing Blocks/motohawk_override_abs  parent_name='LowCellTemp'  parent_val=0  show_more=off  name_source=Use Parameter  parent_read_level=1  parent_override_level=1  view_as=Number  enum_struct={'Disabled', 'Enabled'}  use_help_units=off  parent_help=''  parent_units=''  use_min_max=off  parent_min=-inf  parent_max=inf  use_precision=off  parent_precision=''  parent_gain=1  parent_offset=0  parent_exp=1  use_mototune_group=off  parent_group=motohawk_vardec_path(gcb)
  motohawk_probe : MotoHawk_lib/Calibration & Probing Blocks/motohawk_probe  nam='LowCellTemp'  show_more=off  name_source=Use Parameter  read_level=1  view_as=Number  enum_struct={'Disabled', 'Enabled'}  vector_style=Wide Row  use_help_units=off  help=''  units=''  use_header_enum=off  row_header_enum={}  col_header_enum={}  use_min_max=off  min_val=-inf  max_val=inf  use_precision=off  precision=''  gain=1  offset=0  exp=1  use_mototune_group=off  mototune_group=motohawk_vardec_path(gcb)
  motohawk_probe1 : MotoHawk_lib/Calibration & Probing Blocks/motohawk_probe  nam='HighCellTemp'  show_more=off  name_source=Use Parameter  read_level=1  view_as=Number  enum_struct={'Disabled', 'Enabled'}  vector_style=Wide Row  use_help_units=off  help=''  units=''  use_header_enum=off  row_header_enum={}  col_header_enum={}  use_min_max=off  min_val=-inf  max_val=inf  use_precision=off  precision=''  gain=1  offset=0  exp=1  use_mototune_group=off  mototune_group=motohawk_vardec_path(gcb)
  CellTemps : Outport
  wires:
  Read CAN Message/2 -> Signal Specification1/1
  Read CAN Message/1 -> Signal Specification/1
  Signal Specification1/1 -> motohawk_override_abs1/1, motohawk_probe/1
  Signal Specification/1 -> motohawk_override_abs/1, motohawk_probe1/1
  motohawk_override_abs/1 -> Bus Creator/1  "HighCellTemp"
  motohawk_override_abs1/1 -> Bus Creator/2  "LowCellTemp"
  Bus Creator/1 -> CellTemps/1

== system GTA_PCMFirmware/Function/1 Inputs and Paramaters/CAN/BMS/Pack Size ==
  Bus Creator : BusCreator  Inputs=1
  Read CAN Message : MotoHawk_lib/CAN Blocks/Read CAN Message  nam='BMS_CAN'  bus=-2  msg=CANMSG_FluxPowerCSPackSize  queue=1  slot=''  valid=off  stale=off  labelwires=off
  Signal Specification : SignalSpecification  OutDataTypeStr=uint8
  motohawk_override_abs : MotoHawk_lib/Calibration & Probing Blocks/motohawk_override_abs  parent_name='ParallelStrings'  parent_val=0  show_more=off  name_source=Use Parameter  parent_read_level=1  parent_override_level=1  view_as=Number  enum_struct={'Disabled', 'Enabled'}  use_help_units=off  parent_help=''  parent_units=''  use_min_max=off  parent_min=-inf  parent_max=inf  use_precision=off  parent_precision=''  parent_gain=1  parent_offset=0  parent_exp=1  use_mototune_group=off  parent_group=motohawk_vardec_path(gcb)
  motohawk_probe : MotoHawk_lib/Calibration & Probing Blocks/motohawk_probe  nam='ParallelStrings'  show_more=off  name_source=Use Parameter  read_level=1  view_as=Number  enum_struct={'Disabled', 'Enabled'}  vector_style=Wide Row  use_help_units=off  help=''  units=''  use_header_enum=off  row_header_enum={}  col_header_enum={}  use_min_max=off  min_val=-inf  max_val=inf  use_precision=off  precision=''  gain=1  offset=0  exp=1  use_mototune_group=off  mototune_group=motohawk_vardec_path(gcb)
  PackSize : Outport
  wires:
  Read CAN Message/1 -> Signal Specification/1
  Signal Specification/1 -> motohawk_override_abs/1, motohawk_probe/1
  motohawk_override_abs/1 -> Bus Creator/1  "PackSize"
  Bus Creator/1 -> PackSize/1

== system GTA_PCMFirmware/Function/1 Inputs and Paramaters/Digital/Shifter/ShifterDebug ==
  Shift_out : Inport
  Bus Creator1 : BusCreator
  CompareErr : simulink/Logic and Bit Operations/Compare To Constant  relop===  const=4  OutDataTypeStr=boolean
  CompareF : simulink/Logic and Bit Operations/Compare To Constant  relop===  const=2  OutDataTypeStr=boolean
  CompareN : simulink/Logic and Bit Operations/Compare To Constant  relop===  const=0  OutDataTypeStr=boolean
  CompareR : simulink/Logic and Bit Operations/Compare To Constant  relop===  const=1  OutDataTypeStr=boolean
  dbgShifter : Outport
  wires:
  Bus Creator1/1 -> dbgShifter/1
  Shift_out/1 -> CompareN/1, CompareR/1, CompareF/1, CompareErr/1
  CompareN/1 -> Bus Creator1/1  "dbgShiftN"
  CompareErr/1 -> Bus Creator1/4  "sbgShiftErr"
  CompareF/1 -> Bus Creator1/3  "dbgShiftF"
  CompareR/1 -> Bus Creator1/2  "dbgShiftR"

== system GTA_PCMFirmware/Function/2 Control Loop/Component Controls/Body Control/Defroster ==
  SYSin : Inport
  Bus Creator : BusCreator  Inputs=1
  Bus Selector1 : BusSelector  OutputSignals=BUS.Input Bus.DigitalIn.RearDefrostSw.DefrostSW
  Chart : Stateflow chart  TreatAsAtomicUnit=on
  motohawk_probe : MotoHawk_lib/Calibration & Probing Blocks/motohawk_probe  nam='Defrost_out'  show_more=off  name_source=Use Parameter  read_level=1  view_as=Number  enum_struct={'Disabled', 'Enabled'}  vector_style=Wide Row  use_help_units=off  help=''  units=''  use_header_enum=off  row_header_enum={}  col_header_enum={}  use_min_max=off  min_val=-inf  max_val=inf  use_precision=off  precision=''  gain=1  offset=0  exp=1  use_mototune_group=off  mototune_group=motohawk_vardec_path(gcb)
  Out1 : Outport
  wires:
  Bus Selector1/1 -> Chart/1(Defrost_sw)  "<DefrostSW>"
  Chart/1(Defrost) -> Bus Creator/1, motohawk_probe/1  "Defrost_out_bool"
  Bus Creator/1 -> Out1/1
  SYSin/1 -> Bus Selector1/1

== system GTA_PCMFirmware/Function/2 Control Loop/Component Controls/Body Control/Inter Wiper ==
  SYSin : Inport
  Bus Creator : BusCreator  Inputs=1
  Bus Selector1 : BusSelector  OutputSignals=BUS.Input Bus.AnalogIn.WiperPot.WiperPotPerc,BUS.Input Bus.DigitalIn.WiperSw.WiperSw
  Chart : Stateflow chart  TreatAsAtomicUnit=on
  motohawk_probe : MotoHawk_lib/Calibration & Probing Blocks/motohawk_probe  nam='Wiper_out'  show_more=off  name_source=Use Parameter  read_level=1  view_as=Number  enum_struct={'Disabled', 'Enabled'}  vector_style=Wide Row  use_help_units=off  help=''  units=''  use_header_enum=off  row_header_enum={}  col_header_enum={}  use_min_max=off  min_val=-inf  max_val=inf  use_precision=off  precision=''  gain=1  offset=0  exp=1  use_mototune_group=off  mototune_group=motohawk_vardec_path(gcb)
  Out1 : Outport
  wires:
  SYSin/1 -> Bus Selector1/1
  Bus Selector1/1 -> Chart/1(Pot_position)  "<WiperPotPerc>"
  Bus Creator/1 -> Out1/1
  Chart/1(Wiper_out) -> Bus Creator/1, motohawk_probe/1  "Wiper_out_bool"
  Bus Selector1/2 -> Chart/2(Wiper_Enable)  "<WiperSw>"

== system GTA_PCMFirmware/Function/2 Control Loop/Component Controls/Body Control/Reverse Lights ==
  SYSin : Inport
  MotorControl : Inport  Port=2
  Bus Creator : BusCreator  Inputs=1
  Bus Selector1 : BusSelector  OutputSignals=fndOutput
  Constant : Constant  Value=fndRev
  Relational Operator : RelationalOperator  Operator===  OutDataTypeStr=boolean
  Terminator : Terminator
  Out1 : Outport
  wires:
  SYSin/1 -> Terminator/1
  MotorControl/1 -> Bus Selector1/1
  Bus Creator/1 -> Out1/1
  Bus Selector1/1 -> Relational Operator/1  "<fndOutput>"
  Constant/1 -> Relational Operator/2
  Relational Operator/1 -> Bus Creator/1  "Reverse_out_bool"
